simulink model "simpleMovement"  (R2023a)
settings: Solver=FixedStepAuto  StartTime=0.0  StopTime=inf  RelTol=1e-3
undefined symbols (not defined in the file or in its folder): Levenberg, Marquardt
libraries: robotmaniplib x1, mjLib x1, sharedtransform x1
settings Model: Creator=vmano  LastModifiedBy=vmano
settings OptimizationCC: ReuseModelBlockBuffer=off

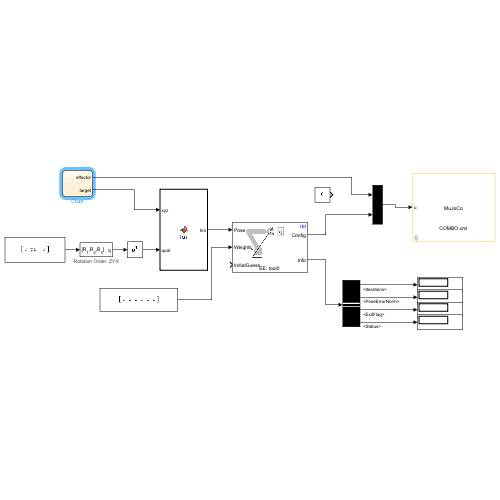
[thumbnail: Simulink's stored preview of the top-level diagram]
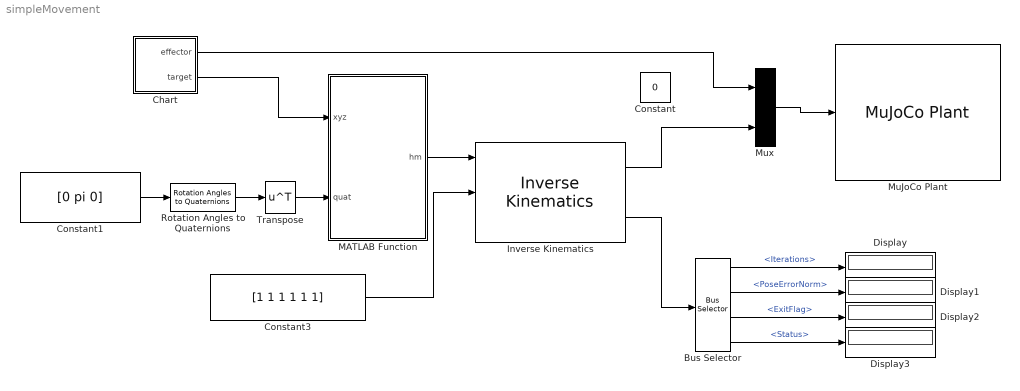
== system simpleMovement ==
  Bus Selector : BusSelector  OutputSignals=Iterations,PoseErrorNorm,ExitFlag,Status
  Chart : Stateflow chart  TreatAsAtomicUnit=on
  Constant : Constant  Value=0
  Constant1 : Constant  Value=[0 pi 0]  VectorParams1D=off
  Constant3 : Constant  Value=[1 1 1 1 1 1]
  Display{,1..3} (4 alike) : Display
  Inverse Kinematics : robotmaniplib/Inverse Kinematics  RigidBodyTree=rbt  EndEffector=tool0  ShowInfo=on  SolverName=Levenberg-Marquardt  EnforceJointLimits=on  MaxIterations=1500  MaxTime=10  GradientTolerance=1e-7  SolutionTolerance=1e-6  StepTolerance=1e-14  ErrorChangeTolerance=1e-12  UseErrorDamping=on  DampingBias=0.0025  SimulateUsing=Code generation
  MATLAB Function : MATLAB Function  TreatAsAtomicUnit=on
  MuJoCo Plant : mjLib/MuJoCo Plant  controlBus=[]  sensorBus=mj_bus_sensor_7979902499018342666  controlLength=[]  sensorLength=[]  rgbLength=[]  depthLength=[]  sampleTime=0.002  xmlFileRel=./models/COMBO.xml  xmlFile=./models/COMBO.xml  renderingType=Global  vsync=off  visualFPS=60  zoomLevel=1  znear=0.02  zfar=100  cameraSampleTime=0.020  rgbOutOption=on  depthOutOption=on  controlInterfaceType=Vector
      settings: SourceProductName=MuJoCo Simulator
  Mux : Mux  Inputs=2
  Rotation Angles to Quaternions : sharedtransform/Rotation Angles to Quaternions  rotationOrder=ZYX  aMode=aMode
  Transpose : Math  Operator=transpose
  wires:
  Mux/1 -> MuJoCo Plant/1
  Inverse Kinematics/1 -> Mux/2
  MATLAB Function/1(hm) -> Inverse Kinematics/1
  Inverse Kinematics/2 -> Bus Selector/1
  Bus Selector/1 -> Display/1  "<Iterations>"
  Bus Selector/2 -> Display1/1  "<PoseErrorNorm>"
  Bus Selector/3 -> Display2/1  "<ExitFlag>"
  Bus Selector/4 -> Display3/1  "<Status>"
  Constant3/1 -> Inverse Kinematics/2
  Constant1/1 -> Rotation Angles to Quaternions/1
  Transpose/1 -> MATLAB Function/2(quat)
  Rotation Angles to Quaternions/1 -> Transpose/1
  Chart/2(target) -> MATLAB Function/1(xyz)
  Chart/1(effector) -> Mux/1

== matlab function simpleMovement/MATLAB Function ==
  data: xyz input; hm output; quat input
function hm = fcn(xyz, quat)
compactpose = zeros(1,7);
hms = zeros(4,4);
compactpose = [xyz, quat];


hms = se3(compactpose, 'xyzquat');

hm = hms.tform;

== stateflow chart simpleMovement/Chart ==
  state init
    en:
    target = [0.5 -0.5 0.2];
    effector = 0;
  state move1
    en:
    effector = 0;
  state move
    en:
    target = [-0.5 -0.5 0.5];
  state object
    en:
    target = [0.5 -0.5 0];
  state pick
    en:
    effector = 200;
  (default) -> init
  move -> move1 : [after(1, sec)]
  init -> object : [after(1, sec)]
  pick -> move : [after(1, sec)]
  object -> pick : [after(1, sec)]
  data: effector output; target output
